simulink model "FileSimulink"  (R2014a)
settings: Solver=ode45  StartTime=0.0  StopTime=100  RelTol=1e-3
libraries: cstblocks x3, simulink x1
settings Model: Creator=User  LastModifiedBy=User

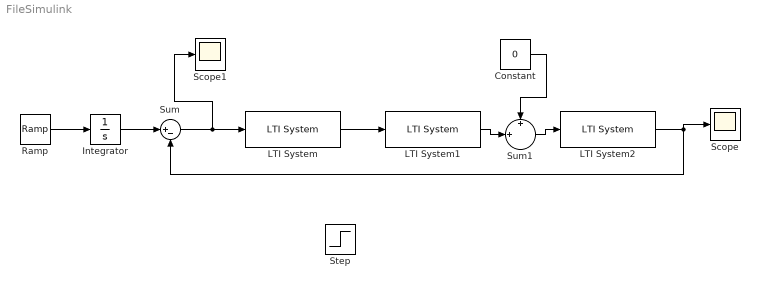
== system FileSimulink ==
  Constant : Constant  Value=0
  Integrator : Integrator
  LTI System : cstblocks/LTI System  sys=C  IC=[]
  LTI System1 : cstblocks/LTI System  sys=F1  IC=[]
  LTI System2 : cstblocks/LTI System  sys=F2  IC=[]
  Ramp : simulink/Sources/Ramp  slope=1  start=0  X0=0
  Scope : Scope
  Scope1 : Scope
  Step : Step  Time=0  SampleTime=0
  Sum : Sum  Inputs=|+-
  Sum1 : Sum  Inputs=+|+||
  wires:
  Sum1/1 -> LTI System2/1
  LTI System1/1 -> Sum1/2
  Constant/1 -> Sum1/1
  LTI System2/1 -> Sum/2, Scope/1
  Sum/1 -> Scope1/1, LTI System/1
  LTI System/1 -> LTI System1/1
  Ramp/1 -> Integrator/1
  Integrator/1 -> Sum/1
